simulink model "receive_blocker_test"  (R2021b)
settings: Solver=VariableStepAuto  StartTime=0.0  StopTime=stop_time-1  RelTol=1e-3
libraries: dspsrcs4 x2
settings Model: Creator=torha  LastModifiedBy=torha
settings SolverCC: AlgebraicLoopSolver=TrustRegion
settings DebuggingCC: SFMachineParentedDataDiag=warning

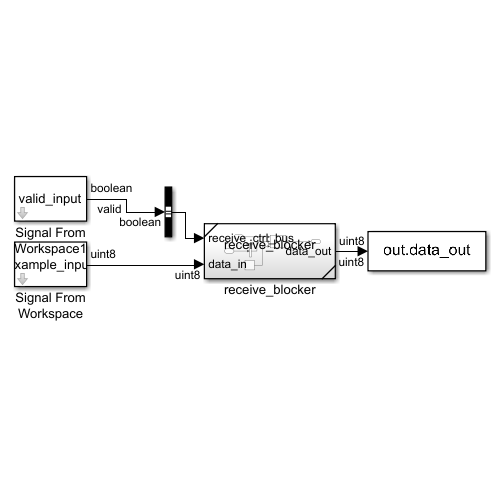
[thumbnail: Simulink's stored preview of the top-level diagram]
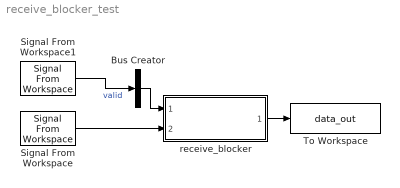
== system receive_blocker_test ==
  Bus Creator : BusCreator  Inputs=1
  Signal From Workspace : dspsrcs4/Signal From Workspace  X=example_input  Ts=1  nsamps=1  OutputAfterFinalValue=Setting to zero  ignoreOrWarnInputAndFrameLengths=off  OutputFrames=off
  Signal From Workspace1 : dspsrcs4/Signal From Workspace  X=valid_input  Ts=1  nsamps=1  OutputAfterFinalValue=Setting to zero  ignoreOrWarnInputAndFrameLengths=off  OutputFrames=off
  To Workspace : ToWorkspace  VariableName=data_out  SampleTime=-1
      settings: Save2DSignal=2-D array (concatenate along first dimension)
  receive_blocker : Subsystem  ReferencedSubsystem=receive_blocker
  wires:
  Signal From Workspace/1 -> receive_blocker/2
  Signal From Workspace1/1 -> Bus Creator/1  "valid"
  receive_blocker/1 -> To Workspace/1
  Bus Creator/1 -> receive_blocker/1
